simulink model "S_MPPT_CONTROLLERS_SIM_V3"  (R2017a)
settings: Solver=VariableStepAuto  StartTime=0.0  StopTime=11  FixedStep=1e-6  MaxStep=1e-4  RelTol=1e-3
values from neighbouring files (symbols this model uses):
  a = 1    [EXPER_PARAMETERS_V1.m]    (also in M_MPPT_CONTROLLERS_SIM_V1.m; TSUKAMOTO_FUZZY_MODEL_V1.m)
  Cload = 470e-6    (= 0.00047)    [M_MPPT_CONTROLLERS_SIM_V1.m]
  Co = 1e-6    (= 1e-06)    [M_MPPT_CONTROLLERS_SIM_V1.m]
  Dmax = Ucmax    (= 9000)    [EXPER_PARAMETERS_V1.m]    (also in M_MPPT_CONTROLLERS_SIM_V1.m = 65535)
  Fred = fs    (= 60)    [M_MPPT_CONTROLLERS_SIM_V1.m]
  fs = 60    [M_MPPT_CONTROLLERS_SIM_V1.m]
  Icc_calc = In/(5/100)    [M_MPPT_CONTROLLERS_SIM_V1.m]
  K1 = K1y2md    [EXPER_PARAMETERS_V1.m]    (also in M_MPPT_CONTROLLERS_SIM_V1.m = K(1:end-1))
  K2 = Kimd    [EXPER_PARAMETERS_V1.m]    (also in M_MPPT_CONTROLLERS_SIM_V1.m = K(end))
  Kh1 = 1/ipv    (= 0.35)    [EXPER_PARAMETERS_V1.m]    (also in M_MPPT_CONTROLLERS_SIM_V1.m = 0.0636345580933)
  KI1 = Kp1/Ti1*Ts1    (= 760)    [EXPER_PARAMETERS_V1.m]    (also in M_MPPT_CONTROLLERS_SIM_V1.m = 95.322582)
  KI2 = Ki2*Ts4    [M_MPPT_CONTROLLERS_SIM_V1.m]
  KI4 = Ki4*Ts4    [M_MPPT_CONTROLLERS_SIM_V1.m]
  KI5 = Ki5*Ts_inv    (= 0.17765287922)    [M_MPPT_CONTROLLERS_SIM_V1.m]
  KP1 = Kp1-KI1/2    (= 5320)    [EXPER_PARAMETERS_V1.m]    (also in M_MPPT_CONTROLLERS_SIM_V1.m = 4107.638709)
  KP2 = Kp2-KI2/2    [M_MPPT_CONTROLLERS_SIM_V1.m]
  KP4 = Kp4-KI4/2    [M_MPPT_CONTROLLERS_SIM_V1.m]
  KP5 = Kp5*Ts_inv-KI5/2    (= -0.0874937760062)    [M_MPPT_CONTROLLERS_SIM_V1.m]
  L = 4.4e-3    (= 0.0044)    [EXPER_PARAMETERS_V1.m]    (also in M_MPPT_CONTROLLERS_SIM_V1.m = 0.100000049318)
  Linv = 0.0133    [M_MPPT_CONTROLLERS_SIM_V1.m]
  Rinv = 0.0417    [M_MPPT_CONTROLLERS_SIM_V1.m]
  S = 10e3*3/2    (= 15000)    [M_MPPT_CONTROLLERS_SIM_V1.m]
  Ts1 = 1/Fs    (= 0.0002)    [EXPER_PARAMETERS_V1.m]    (also in M_MPPT_CONTROLLERS_SIM_V1.m)
  Ts3 = Ts1    (= 0.0002)    [EXPER_PARAMETERS_V1.m]    (also in M_MPPT_CONTROLLERS_SIM_V1.m; TSUKAMOTO_FUZZY_MODEL_V1.m)
  Ts4 = 1/(4*Fc)    (= 0.000125)    [M_MPPT_CONTROLLERS_SIM_V1.m]
  Ts_inv = 1/(100*Fc)    (= 5e-06)    [M_MPPT_CONTROLLERS_SIM_V1.m]
  Univ_discurso = 0.015*1    (= 0.015)    [EXPER_PARAMETERS_V1.m]    (also in M_MPPT_CONTROLLERS_SIM_V1.m; TSUKAMOTO_FUZZY_MODEL_V1.m)
  vdc = 12    [EXPER_PARAMETERS_V1.m]    (also in M_MPPT_CONTROLLERS_SIM_V1.m = 1000)
  vdc_ref = vdc    (= 12)    [EXPER_PARAMETERS_V1.m]    (also in M_MPPT_CONTROLLERS_SIM_V1.m = 1000)
  Vf = VL/sqrt(3)    [M_MPPT_CONTROLLERS_SIM_V1.m]
  VL = (381.051/2)    (= 190.5255)    [M_MPPT_CONTROLLERS_SIM_V1.m]
undefined symbols (not defined in the file or in its folder): DiscIntNeverNeededParam, sigbuilder_block
undefined symbols (not defined in the file): Fs
libraries: powerlib x22, powerlib_meascontrol x10, simulink x7, fuzblock x4, dsparch4 x3, re_lib x1
(part 2 of 2)

== system S_MPPT_CONTROLLERS_SIM_V3/A Measurements/n_mppt (%) ==
  note: time < 0.01 para curve
      | time < 0.201 para steps
  note: Init cond 1 para steps y hab ext resett
  note: Init cond 0 para steps y hab ext reset
  In1 : Inport
  In2 : Inport  Port=2
  Clock : Clock
  Divide : Product  Inputs=/*
  Gain : Gain  Gain=100
  Integrator1 : Integrator  ExternalReset=level hold  InitialCondition=1  ZeroCross=off
  Integrator2 : Integrator  ExternalReset=level hold  ZeroCross=off
  MATLAB Function : MATLAB Function  TreatAsAtomicUnit=on
  Out1 : Outport
  tag scope: Pvkwh=global
  wires:
  In2/1 -> Integrator2/1
  Gain/1 -> Out1/1
  In1/1 -> Integrator1/1
  Integrator1/1 -> Divide/1
  Integrator2/1 -> [Pvkwh], Divide/2
  Divide/1 -> Gain/1
  Clock/1 -> MATLAB Function/1(time)
  MATLAB Function/1(y) -> Integrator1/2, Integrator2/2

== system S_MPPT_CONTROLLERS_SIM_V3/DPWM/Modulation Carrier ==
  Clock : Clock
  Fcn : Fcn  Expr=u*fc-offset
  Lookup Table : Lookup  InputValues=[0 .5 1]  Table=[range(1) range(2) range(1)]  LookUpMeth=Interpolation-Use End Values
  Rounding Function : Rounding
  Subtract : Sum  Inputs=+-
  Unit Delay : UnitDelay  SampleTime=si
  Out : Outport
  wires:
  Lookup Table/1 -> Out/1
  Subtract/1 -> Lookup Table/1
  Rounding Function/1 -> Subtract/2
  Fcn/1 -> Rounding Function/1, Subtract/1
  Clock/1 -> Fcn/1
  Unit Delay/1 -> Unit Delay/1

== matlab function S_MPPT_CONTROLLERS_SIM_V3/Digital PI Current Controller n_mppt = 97.81%, ta(2%) = 0.5 s con Steps de Irrad Interv. 2 Seg. n_mppt = 98.24%, ta(2%) = 0.4 s con Steps de Irrad Interv. 2 Seg. n_mppt = 98.7%, ta(2%) = 0.25 s con Steps de Irrad Interv. 2 Seg. n_mppt = 91.8%, ta(2%) = 0.5 s con Steps de Irrad Interv. 0.5 Seg. n_mppt = 93.49%, ta(2%) = 0.4 s con Steps de Irrad Interv. 0.5 Seg. n_mppt = 95.28%, ta(2%) = 0.25 s con Steps de Irrad Interv. 0.5 Seg. n_mppt = 97.87%, ta(2%) = 0.25 s con Curva de Irrad ta(2%) de 0.25 s se obtiene el ta de F-Tsukmam Menor ta y tr: mayor n_mppt pero genera mayor MP en id (impacto negativo PQ) en el punto de operación  (15.71 A). Si se mantiene ta y se incrementa tr la n_mppt se mantiene al mismo tiempo que se mitigan los MP en id (impacto positivo en PQ) /PID Digital I 1 ==
  data: In_ref input; UK output; In input; KI input; KP input
function UK = fcn(In_ref, In, KI, KP)

 %Valores iniciales de las conStantes del controlador
 persistent  ek uk
 persistent  ek_1 uk_1
 if isempty(ek)
    ek =0;
    uk =0;
    ek_1 =0;
    uk_1 =0;
 end
ek=In_ref-In;
uk=ek*(KP+KI)-ek_1*KP+uk_1;
%uk=KP*ek+KI*ek+KI*ek_1;
if(uk>(1*65535))
    uk=1*65535;
end
if(uk<0)
    uk=0;
end
ek_1=ek;
uk_1=uk;
UK=uk;
end

== matlab function S_MPPT_CONTROLLERS_SIM_V3/ DQ control/PID Digital I 1 ==
  data: IN_ref input; UK output; IN input; KI input; KP input
function UK = fcn(IN_ref, IN, KI, KP)

 %Valores iniciales de las conStantes del controlador
 persistent  ek uk
 persistent  ek_1 uk_1
 if isempty(ek)
    ek =0;
    uk =0;
    ek_1 =0;
    uk_1 =0;
 end
ek=IN_ref-IN;
uk=ek*(KP+KI)-ek_1*KP+uk_1;
if(uk>1000)
    uk=1000;
end
if(uk<-1000)
    uk=-1000;
end
ek_1=ek;
uk_1=uk;
UK=uk;
end

== matlab function S_MPPT_CONTROLLERS_SIM_V3/ DQ control/PID Digital I 2 ==
  data: IN_ref input; UK output; IN input; KI input; KP input
function UK = fcn(IN_ref, IN, KI, KP)

 %Valores iniciales de las conStantes del controlador
 persistent  ek uk
 persistent  ek_1 uk_1
 if isempty(ek)
    ek =0;
    uk =0;
    ek_1 =0;
    uk_1 =0;
 end
ek=IN_ref-IN;
uk=ek*(KP+KI)-ek_1*KP+uk_1;
if(uk>1000)
    uk=1000;
end
if(uk<-1000)
    uk=-1000;
end
ek_1=ek;
uk_1=uk;
UK=uk;
end

== matlab function S_MPPT_CONTROLLERS_SIM_V3/ DQ control/PID Digital I 3 ==
  data: IN_ref input; UK output; IN input; KI input; KP input
function UK = fcn(IN_ref, IN, KI, KP)

 %Valores iniciales de las conStantes del controlador
 persistent  ek uk
 persistent  ek_1 uk_1
 if isempty(ek)
    ek =0;
    uk =0;
    ek_1 =0;
    uk_1 =0;
 end
ek=IN_ref-IN;
uk=ek*(KP+KI)-ek_1*KP+uk_1;
if(uk>60)
    uk=60;
end
if(uk<-60)
    uk=-60;
end
ek_1=ek;
uk_1=uk;
UK=uk;
end

== matlab function S_MPPT_CONTROLLERS_SIM_V3/PLL/PID Digital I 7 ==
  data: Ref input; Out output; Med input; KI input; KP input
function Out = fcn(Ref, Med, KI, KP)

 %Valores iniciales de las conStantes del controlador
 persistent  ek uk
 persistent  ek_1 uk_1
 if isempty(ek)
    ek =0;
    uk =0;
    ek_1 =0;
    uk_1 =0;
 end
ek=Ref-Med;
%uk=ek*(KP+KI)-ek_1*KP+uk_1;
uk=KP*ek+KI*ek+KI*ek_1;
ek_1=ek;
uk_1=uk;
Out=uk;
end

== matlab function S_MPPT_CONTROLLERS_SIM_V3/Fuzzy Tsukamoto Current Controller n_mppt = 99.11%, ta(2%) = 0.12 s con Steps de Irrad Interv. 2 Seg. n_mppt = 96.74%, ta(2%) = 0.12 s con Steps de Irrad Interv. 0.5 Seg. n_mppt = 99.37%, ta(2%) = 0.12 s con Curva de Irrad Este controlador puede disminuir ta e incrementar a tr para mitigar los MP en id (impacto positivo en PQ) /Linear combination ==
  data: mA1 input; y0 output; mA2 input; Adj input; UD input
function y0 = fcn(mA1,mA2,Adj, UD)
w1=mA1;
w2=mA2;
z1 = -(UD)*(w1-0.5);
z2 = (UD)*(w2-0.5);
y0 = ((w1*z1 + w2*z2)/(w1+w2))+Adj;
end

== matlab function S_MPPT_CONTROLLERS_SIM_V3/Digital State Feedback Current Controller n_mppt = 88.18%, ta(2%) = 0.4 s con Steps de Irrad Interv. 2 Seg. n_mppt = 97.01%, ta(2%) = 0.1 s con Steps de Irrad Interv. 2 Seg. n_mppt = 86.2%, ta(2%) = 0.4 s con Steps de Irrad Interv. 0.5 Seg. n_mppt = 93.3%, ta(2%) = 0.1 s con Steps de Irrad Interv. 0.5 Seg. n_mppt = 96.15%, ta(2%) = 0.1 s con Curva de Irrad ta(2%) de 0.1 s se obtiene el ta de F-Tsukmam n_mppt = 89.31%, ta(2%) = 0.0692 s con Steps de Irrad Interv. 0.5 Seg. Menor ta y tr: mayor n_mppt pero genera mayor MP en id (impacto negativo PQ). Si se mantiene ta y se incrementa tr la n_mppt se mantiene al mismo tiempo que se mitigan los MP en id (impacto positivo en PQ)  /PID Digital I 2 ==
  data: iL_ref input; iL input; UK output; vdc input; KI input; K1 input; K2 input
function UK = fcn(iL_ref, iL, vdc, KI, K1, K2)

 %Valores iniciales de las conStantes del controlador
 persistent  ek Acc_Int uk
 persistent  Acc_Int_1
 if isempty(ek)
    ek =0;
    uk =0;
    Acc_Int =0;
    Acc_Int_1 =0;
 end
ek=iL_ref- iL;
Acc_Int=ek*KI+Acc_Int_1;
Acc_Int_1=Acc_Int;
uk=Acc_Int-(K1*iL+K2*vdc);
if(uk>(1*65535))
    uk=1*65535;
end
if(uk<0)
    uk=0;
end
UK=uk;
end

== matlab function S_MPPT_CONTROLLERS_SIM_V3/A Measurements/n_mppt (%)/MATLAB Function ==
  data: y output; time input
function y = fcn(time)
    % Verifica si el valor es Inf
    if time < 0.201
        y = 1;  % Si es Inf, asigna 0
    else
        y = 0;  % Si no es Inf, devuelve el valor original
    end
end

== matlab function S_MPPT_CONTROLLERS_SIM_V3/A Measurements/MATLAB Function ==
  data: u input; sigma_d output; t input
function sigma_d = fcn(u,t)

persistent n sum_u sum_u2 sigma_last

if isempty(n)
    n = 0;
    sum_u = 0;
    sum_u2 = 0;
    sigma_last = 0;
end

% Acumular muestras de d únicamente entre 1.5 y 2.9 s
if (t >= 1.5) && (t <= 2.9)
    n = n + 1;
    sum_u = sum_u + u;
    sum_u2 = sum_u2 + u*u;
end

% Calcular la desviación estándar muestral
if n > 1
    variance = (sum_u2 - (sum_u*sum_u)/n)/(n - 1);

    % Evitar valores negativos pequeños por redondeo numérico
    if variance < 0
        variance = 0;
    end

    sigma_last = sqrt(variance);
end

% Salida en unidades normalizadas de duty cycle
sigma_d = 100*sigma_last;

end

== matlab function S_MPPT_CONTROLLERS_SIM_V3/Noise/MATLAB Function ==
  data: u input; y output
function y = fcn(u)

Gmin = 50;   % W/m^2

if u < Gmin
    y = 0;
else
    y = u;
end

== matlab function S_MPPT_CONTROLLERS_SIM_V3/Fuzzy Tsukamoto Current Controller n_mppt = 99.11%, ta(2%) = 0.12 s con Steps de Irrad Interv. 2 Seg. n_mppt = 96.74%, ta(2%) = 0.12 s con Steps de Irrad Interv. 0.5 Seg. n_mppt = 99.37%, ta(2%) = 0.12 s con Curva de Irrad Este controlador puede disminuir ta e incrementar a tr para mitigar los MP en id (impacto positivo en PQ) /MATLAB Function ==
  data: x input; y output
function y = fcn(x)

% Low-pass filter for irradiance

Ts = 1/5000;
fc = 50;          % Hz
a  = 2*pi*fc;

persistent yk

if isempty(yk)
    yk = x;
end

yk = (yk + Ts*a*x)/(1 + Ts*a);

y = yk;

== matlab function S_MPPT_CONTROLLERS_SIM_V3/Fuzzy Tsukamoto Current Controller n_mppt = 99.11%, ta(2%) = 0.12 s con Steps de Irrad Interv. 2 Seg. n_mppt = 96.74%, ta(2%) = 0.12 s con Steps de Irrad Interv. 0.5 Seg. n_mppt = 99.37%, ta(2%) = 0.12 s con Curva de Irrad Este controlador puede disminuir ta e incrementar a tr para mitigar los MP en id (impacto positivo en PQ) /MATLAB Function1 ==
  data: x input; y output
function y = fcn(x)

% Low-pass filter for input current

Ts = 1/5000;
fc = 50;          % Hz
a  = 2*pi*fc;

persistent yk

if isempty(yk)
    yk = x;
end

yk = (yk + Ts*a*x)/(1 + Ts*a);

y = yk;

== matlab function S_MPPT_CONTROLLERS_SIM_V3/Digital PI Current Controller n_mppt = 97.81%, ta(2%) = 0.5 s con Steps de Irrad Interv. 2 Seg. n_mppt = 98.24%, ta(2%) = 0.4 s con Steps de Irrad Interv. 2 Seg. n_mppt = 98.7%, ta(2%) = 0.25 s con Steps de Irrad Interv. 2 Seg. n_mppt = 91.8%, ta(2%) = 0.5 s con Steps de Irrad Interv. 0.5 Seg. n_mppt = 93.49%, ta(2%) = 0.4 s con Steps de Irrad Interv. 0.5 Seg. n_mppt = 95.28%, ta(2%) = 0.25 s con Steps de Irrad Interv. 0.5 Seg. n_mppt = 97.87%, ta(2%) = 0.25 s con Curva de Irrad ta(2%) de 0.25 s se obtiene el ta de F-Tsukmam Menor ta y tr: mayor n_mppt pero genera mayor MP en id (impacto negativo PQ) en el punto de operación  (15.71 A). Si se mantiene ta y se incrementa tr la n_mppt se mantiene al mismo tiempo que se mitigan los MP en id (impacto positivo en PQ) /MATLAB Function ==
  data: x input; y output
function y = fcn(x)

% Low-pass filter for irradiance

Ts = 1/5000;
fc = 50;          % Hz
a  = 2*pi*fc;

persistent yk

if isempty(yk)
    yk = x;
end

yk = (yk + Ts*a*x)/(1 + Ts*a);

y = yk;

== matlab function S_MPPT_CONTROLLERS_SIM_V3/Digital PI Current Controller n_mppt = 97.81%, ta(2%) = 0.5 s con Steps de Irrad Interv. 2 Seg. n_mppt = 98.24%, ta(2%) = 0.4 s con Steps de Irrad Interv. 2 Seg. n_mppt = 98.7%, ta(2%) = 0.25 s con Steps de Irrad Interv. 2 Seg. n_mppt = 91.8%, ta(2%) = 0.5 s con Steps de Irrad Interv. 0.5 Seg. n_mppt = 93.49%, ta(2%) = 0.4 s con Steps de Irrad Interv. 0.5 Seg. n_mppt = 95.28%, ta(2%) = 0.25 s con Steps de Irrad Interv. 0.5 Seg. n_mppt = 97.87%, ta(2%) = 0.25 s con Curva de Irrad ta(2%) de 0.25 s se obtiene el ta de F-Tsukmam Menor ta y tr: mayor n_mppt pero genera mayor MP en id (impacto negativo PQ) en el punto de operación  (15.71 A). Si se mantiene ta y se incrementa tr la n_mppt se mantiene al mismo tiempo que se mitigan los MP en id (impacto positivo en PQ) /MATLAB Function1 ==
  data: x input; y output
function y = fcn(x)

% Low-pass filter for input current

Ts = 1/5000;
fc = 50;          % Hz
a  = 2*pi*fc;

persistent yk

if isempty(yk)
    yk = x;
end

yk = (yk + Ts*a*x)/(1 + Ts*a);

y = yk;

== matlab function S_MPPT_CONTROLLERS_SIM_V3/Fuzzy Mamdani Current Controller n_mppt = 98.87%, ta(2%) = 0.12 s con Steps de Irrad Interv. 2 Seg. n_mppt = 95.78%, ta(2%) = 0.12 s con Steps de Irrad Interv. 0.5 Seg. n_mppt = 98.21%, ta(2%) = 0.12 s con Curva de Irrad/MATLAB Function ==
  data: x input; y output
function y = fcn(x)

% Low-pass filter for irradiance

Ts = 1/5000;
fc = 50;          % Hz
a  = 2*pi*fc;

persistent yk

if isempty(yk)
    yk = x;
end

yk = (yk + Ts*a*x)/(1 + Ts*a);

y = yk;

== matlab function S_MPPT_CONTROLLERS_SIM_V3/Fuzzy Mamdani Current Controller n_mppt = 98.87%, ta(2%) = 0.12 s con Steps de Irrad Interv. 2 Seg. n_mppt = 95.78%, ta(2%) = 0.12 s con Steps de Irrad Interv. 0.5 Seg. n_mppt = 98.21%, ta(2%) = 0.12 s con Curva de Irrad/MATLAB Function1 ==
  data: x input; y output
function y = fcn(x)

% Low-pass filter for input current

Ts = 1/5000;
fc = 50;          % Hz
a  = 2*pi*fc;

persistent yk

if isempty(yk)
    yk = x;
end

yk = (yk + Ts*a*x)/(1 + Ts*a);

y = yk;

== matlab function S_MPPT_CONTROLLERS_SIM_V3/Fuzzy Tsukamoto Current Controller n_mppt = 99.11%, ta(2%) = 0.12 s con Steps de Irrad Interv. 2 Seg. n_mppt = 96.74%, ta(2%) = 0.12 s con Steps de Irrad Interv. 0.5 Seg. n_mppt = 99.37%, ta(2%) = 0.12 s con Curva de Irrad Este controlador puede disminuir ta e incrementar a tr para mitigar los MP en id (impacto positivo en PQ) 1/MATLAB Function2 ==
  data: x input; y output
function y = fcn(x)

% Low-pass filter for input current

Ts = 1/5000;
fc = 50;          % Hz
a  = 2*pi*fc;

persistent yk

if isempty(yk)
    yk = x;
end

yk = (yk + Ts*a*x)/(1 + Ts*a);

y = yk;

== matlab function S_MPPT_CONTROLLERS_SIM_V3/Fuzzy Tsukamoto Current Controller n_mppt = 99.11%, ta(2%) = 0.12 s con Steps de Irrad Interv. 2 Seg. n_mppt = 96.74%, ta(2%) = 0.12 s con Steps de Irrad Interv. 0.5 Seg. n_mppt = 99.37%, ta(2%) = 0.12 s con Curva de Irrad Este controlador puede disminuir ta e incrementar a tr para mitigar los MP en id (impacto positivo en PQ) 1/MATLAB Function1 ==
  data: x input; y output
function y = fcn(x)

% Low-pass filter for input current

Ts = 1/5000;
fc = 50;          % Hz
a  = 2*pi*fc;

persistent yk

if isempty(yk)
    yk = x;
end

yk = (yk + Ts*a*x)/(1 + Ts*a);

y = yk;

== matlab function S_MPPT_CONTROLLERS_SIM_V3/Digital State Feedback Current Controller n_mppt = 88.18%, ta(2%) = 0.4 s con Steps de Irrad Interv. 2 Seg. n_mppt = 97.01%, ta(2%) = 0.1 s con Steps de Irrad Interv. 2 Seg. n_mppt = 86.2%, ta(2%) = 0.4 s con Steps de Irrad Interv. 0.5 Seg. n_mppt = 93.3%, ta(2%) = 0.1 s con Steps de Irrad Interv. 0.5 Seg. n_mppt = 96.15%, ta(2%) = 0.1 s con Curva de Irrad ta(2%) de 0.1 s se obtiene el ta de F-Tsukmam n_mppt = 89.31%, ta(2%) = 0.0692 s con Steps de Irrad Interv. 0.5 Seg. Menor ta y tr: mayor n_mppt pero genera mayor MP en id (impacto negativo PQ). Si se mantiene ta y se incrementa tr la n_mppt se mantiene al mismo tiempo que se mitigan los MP en id (impacto positivo en PQ)  /MATLAB Function ==
  data: x input; y output
function y = fcn(x)

% Low-pass filter for irradiance

Ts = 1/5000;
fc = 50;          % Hz
a  = 2*pi*fc;

persistent yk

if isempty(yk)
    yk = x;
end

yk = (yk + Ts*a*x)/(1 + Ts*a);

y = yk;

== matlab function S_MPPT_CONTROLLERS_SIM_V3/Digital State Feedback Current Controller n_mppt = 88.18%, ta(2%) = 0.4 s con Steps de Irrad Interv. 2 Seg. n_mppt = 97.01%, ta(2%) = 0.1 s con Steps de Irrad Interv. 2 Seg. n_mppt = 86.2%, ta(2%) = 0.4 s con Steps de Irrad Interv. 0.5 Seg. n_mppt = 93.3%, ta(2%) = 0.1 s con Steps de Irrad Interv. 0.5 Seg. n_mppt = 96.15%, ta(2%) = 0.1 s con Curva de Irrad ta(2%) de 0.1 s se obtiene el ta de F-Tsukmam n_mppt = 89.31%, ta(2%) = 0.0692 s con Steps de Irrad Interv. 0.5 Seg. Menor ta y tr: mayor n_mppt pero genera mayor MP en id (impacto negativo PQ). Si se mantiene ta y se incrementa tr la n_mppt se mantiene al mismo tiempo que se mitigan los MP en id (impacto positivo en PQ)  /MATLAB Function1 ==
  data: x input; y output
function y = fcn(x)

% Low-pass filter for input current

Ts = 1/5000;
fc = 50;          % Hz
a  = 2*pi*fc;

persistent yk

if isempty(yk)
    yk = x;
end

yk = (yk + Ts*a*x)/(1 + Ts*a);

y = yk;

== matlab function S_MPPT_CONTROLLERS_SIM_V3/Digital State Feedback Current Controller n_mppt = 88.18%, ta(2%) = 0.4 s con Steps de Irrad Interv. 2 Seg. n_mppt = 97.01%, ta(2%) = 0.1 s con Steps de Irrad Interv. 2 Seg. n_mppt = 86.2%, ta(2%) = 0.4 s con Steps de Irrad Interv. 0.5 Seg. n_mppt = 93.3%, ta(2%) = 0.1 s con Steps de Irrad Interv. 0.5 Seg. n_mppt = 96.15%, ta(2%) = 0.1 s con Curva de Irrad ta(2%) de 0.1 s se obtiene el ta de F-Tsukmam n_mppt = 89.31%, ta(2%) = 0.0692 s con Steps de Irrad Interv. 0.5 Seg. Menor ta y tr: mayor n_mppt pero genera mayor MP en id (impacto negativo PQ). Si se mantiene ta y se incrementa tr la n_mppt se mantiene al mismo tiempo que se mitigan los MP en id (impacto positivo en PQ)  /MATLAB Function2 ==
  data: x input; y output
function y = fcn(x)

% Low-pass filter for input current

Ts = 1/5000;
fc = 50;          % Hz
a  = 2*pi*fc;

persistent yk

if isempty(yk)
    yk = x;
end

yk = (yk + Ts*a*x)/(1 + Ts*a);

y = yk;

== matlab function S_MPPT_CONTROLLERS_SIM_V3/A Measurements/MATLAB Function1 ==
  data: u input; sigma_e output; t input
function sigma_e = fcn(u,t)

persistent n sum_u sum_u2 sigma_last

if isempty(n)
    n = 0;
    sum_u = 0;
    sum_u2 = 0;
    sigma_last = 0;
end

% Acumular muestras de d únicamente entre 1.5 y 2.9 s
if (t >= 1.5) && (t <= 2.9)
    n = n + 1;
    sum_u = sum_u + u;
    sum_u2 = sum_u2 + u*u;
end

% Calcular la desviación estándar muestral
if n > 1
    variance = (sum_u2 - (sum_u*sum_u)/n)/(n - 1);

    % Evitar valores negativos pequeños por redondeo numérico
    if variance < 0
        variance = 0;
    end

    sigma_last = sqrt(variance);
end

% Salida en unidades normalizadas de duty cycle
sigma_e = 100*sigma_last;

end

== matlab function S_MPPT_CONTROLLERS_SIM_V3/A Measurements/MATLAB Function2 ==
  data: u input; sigma_iin output; t input
function sigma_iin = fcn(u,t)

persistent n sum_u sum_u2 sigma_last

if isempty(n)
    n = 0;
    sum_u = 0;
    sum_u2 = 0;
    sigma_last = 0;
end

% Acumular muestras de d únicamente entre 1.5 y 2.9 s
if (t >= 1.5) && (t <= 2.9)
    n = n + 1;
    sum_u = sum_u + u;
    sum_u2 = sum_u2 + u*u;
end

% Calcular la desviación estándar muestral
if n > 1
    variance = (sum_u2 - (sum_u*sum_u)/n)/(n - 1);

    % Evitar valores negativos pequeños por redondeo numérico
    if variance < 0
        variance = 0;
    end

    sigma_last = sqrt(variance);
end

% Salida en unidades normalizadas de duty cycle
sigma_iin = 100*sigma_last;

end
